simulink model "Final_Model_Building_2_AirflowAdded"  (R2022a)
settings: Solver=ode1  StartTime=0.0  StopTime=24*3600  FixedStep=10  RelTol=1e-3
values from neighbouring files (symbols this model uses):
  Aux_Threshold = 52    [Setup_Code_EWASP_VC.m]
  buildingAge = 2005    [Setup_Code_EWASP_VC.m]
  ceilingHeight = 2.4    [Setup_Code_EWASP_VC.m]
  conductiveHconnectMatrix = [ ... (first row only)    [Setup_Code_EWASP_VC.m]
  cRoofGreen = 100000    [Setup_Code_EWASP_VC.m]
  Defrost_After_Time = 30    [Setup_Code_EWASP_VC.m]
  DHWDemandProfile = occFreegainHotwaterElecTestPassiveOcc3(:,3)    [Setup_Code_EWASP_VC.m]
  Elec_Max = Elec_Max*(30/24.2)    [Setup_Code_EWASP_VC.m]
  Elec_Mid = Elec_Mid*(30/24.2)    [Setup_Code_EWASP_VC.m]
  Elec_Min = Elec_Min*(30/24.2)    [Setup_Code_EWASP_VC.m]
  ElecDemandProfile = occFreegainHotwaterElecTestPassiveOcc3(:,4)    [Setup_Code_EWASP_VC.m]
  ElecFixed = [Elec_Max(6,2) Elec_Max(6,4) Elec_Max(6,6) Elec_Max(6,7) ... (first row only)    [Setup_Code_EWASP_VC.m]
  floorOrCeilingArea = floorOrCeilingArea*1.15    [Setup_Code_EWASP_VC.m]
  forceCold = 0    [Setup_Code_EWASP_VC.m]
  freegain = occFreegainHotwaterElecTestPassiveOcc3(:,2)-max(occupancy)*25    [Setup_Code_EWASP_VC.m]
  furnitureModelOn = 1    [Setup_Code_EWASP_VC.m]
  Heat_Max = Heat_Max*(30/24.2)    [Setup_Code_EWASP_VC.m]
  Heat_Mid = Heat_Mid*(30/24.2)    [Setup_Code_EWASP_VC.m]
  Heat_Min = Heat_Min*(30/24.2)    [Setup_Code_EWASP_VC.m]
  HeatFixed = [Heat_Max(6,2) Heat_Max(6,4) Heat_Max(6,6) Heat_Max(6,7) ... (first row only)    [Setup_Code_EWASP_VC.m]
  HeatingOnProfile = repmat(HeatingOnProfile,365,1)    [Setup_Code_EWASP_VC.m]
  HEX_ReturnLowerLimit = 52.5    [Setup_Code_EWASP_VC.m]
  HEX_ReturnUpperLimit = 55    [Setup_Code_EWASP_VC.m]
  LeakMultiplier = 1+(2*(rand()-0.5)/10)    [Setup_Code_EWASP_VC.m]
  maxOcc = max(occupancyProfile)    [Setup_Code_EWASP_VC.m]
  NESW_wallArea = max(NESW_Lengths*ceilingHeight-NESW_Windows,0)    [Setup_Code_EWASP_VC.m]
  NESW_Windows = [ ... (first row only)    [Setup_Code_EWASP_VC.m]
  numRooms = roomCount    [Setup_Code_EWASP_VC.m]
  occupancy = occupancyProfile    [Setup_Code_EWASP_VC.m]
  offsetDays = 0    [Setup_Code_EWASP_VC.m]
  pumpChoice = pumpChoices(MinIndex,1)    [Setup_Code_EWASP_VC.m]
  pumpRamp = 180    [Setup_Code_EWASP_VC.m]
  ReturnLowerLimit = 37.5    [Setup_Code_EWASP_VC.m]
  ReturnUpperLimit = 40    [Setup_Code_EWASP_VC.m]
  RoofIrradiance = Flat_NS_EW_RoofIrradiance(:,1)    [Setup_Code_EWASP_VC.m]
  roofStartTemp = ones(11,1)*20    [Setup_Code_EWASP_VC.m]
  rooftype = 0    [Setup_Code_EWASP_VC.m]
  RoomDataMatrix = [zeros(1,12);ones(1,12)*wallDensity;zeros(1,12);ones(1,12)*wallU;ones(1,12)*windowU;ones(1,12)*floorU;ones(1,12)*ceilingU;zeros(1,12);windowArea, 0;floorOrCeilingArea;zeros(1,12);floorOrCeilingArea*ceilingHeight]    [Setup_Code_EWASP_VC.m]
  roomVol = roomVol*1.15    [Setup_Code_EWASP_VC.m]
  slabStartTemp = (GroundTempTimeSeries(offsetDays*1440+1,1)+thermostatSetting)/2    [Setup_Code_EWASP_VC.m]
  SlackRequest = zeros(1440,1)    [Setup_Code_EWASP_VC.m]
  SolarThermalExists = 0    [Setup_Code_EWASP_VC.m]
  SourceFixed = HeatFixed-ElecFixed    [Setup_Code_EWASP_VC.m]
  StateSeries = StateSeriesGenerator(22,7,1)    [Setup_Code_EWASP_VC.m]
  Tank_Lower_Temp = 49.5    [Setup_Code_EWASP_VC.m]
  Tank_Upper_Temp = 52    [Setup_Code_EWASP_VC.m]
  Tank_Volume_m3 = 0.15    [Setup_Code_EWASP_VC.m]
  TankHeatHour = randi([1 5])-1    [Setup_Code_EWASP_VC.m]
  upDown = [0;0;0;0;1;1;1;1;1;1;1]    [Setup_Code_EWASP_VC.m]
  wallStartTempExt = thermostatSetting*(0.266+0.00215*outdoorStartTemp+0.018*wallU+0.00113*outdoorStartTemp*wallU+0.0068*wallU^2)    [Setup_Code_EWASP_VC.m]
undefined symbols (not defined in the file or in its folder): a, ceilingU, condUDMatrix, convUDMatrix, deltaPEXPANDED_E, deltaPEXPANDED_E2, deltaPEXPANDED_N, deltaPEXPANDED_N2, deltaPEXPANDED_S, deltaPEXPANDED_S2, deltaPEXPANDED_W, deltaPEXPANDED_W2, DesiredDHWTemp, DesiredFlowTempVsInOutDeltaTemp, DiffuseHorizontal, DiscIntNeverNeededParam, DNI, dwnAndConcrete, DWORK_A_HX, DWORK_CHK_FLU, DWORK_CP_NODE, DWORK_DH, DWORK_FLUID, DWORK_HCON, DWORK_LOSS, DWORK_MDOTDOWN, DWORK_MDOTIN, DWORK_MDOTUP, DWORK_MIX, DWORK_PRESS, DWORK_QDOTIN, DWORK_RHO_NODE, DWORK_TIN, DWORK_TS_OLD, DWORK_V_NODE, ExtractRates, GroundTempTimeSeries, HCM, HCM2, HCM_closed, HCM_closed2, intermediateU, IsTop, massFlowMatrix, mechEfficiency, neighbourMatrix, numericalRoomUse, RadiatorMatrix, room2roomflowmatrix_E, room2roomflowmatrix_E2, room2roomflowmatrix_N, room2roomflowmatrix_N2, room2roomflowmatrix_S, room2roomflowmatrix_S2, room2roomflowmatrix_W, room2roomflowmatrix_W2, StateAirInEXPANDED_E, StateAirInEXPANDED_E2, StateAirInEXPANDED_N, StateAirInEXPANDED_N2 ... (+27)
libraries: simulink x6, dspsigops x4, dspmtrx3 x4, carnot x3, spsEdgeDetectorLib x2, dspstat3 x2, powerlib_meascontrol x1, simulink_extras x1
(part 12 of 27)

== system Final_Model_Building_2_AirflowAdded/ASHP_Subsystem/DHW for ASHP Case/Storage_Type_2_CONF ==
  note: upper heat exchanger (backup heater)
  note: pipe connection for DHW
  note: pipe connection for DHW circulation
  Tamb : Inport
  Temp_HX : Inport  Port=2
  THB_dhw : Inport  Port=3
  THB_circ : Inport  Port=4
  Mdot_dhw1 : Inport  Port=5
  Mdot_dhw2 : Inport  Port=6
  mdotHEX : Inport  Port=7
  HX_EN12977_1 : Subsystem  AncestorBlock=carnot/Storage/Thermal/Storage_Ports/HX_EN12977  mask(heat exchanger for storage, data EN 12977){h_in=hx1inlet, h_out=hx1outlet, hgt=hgt, dia=hx1dia, height=-0.68756, ua0=hx1uac, uam=hx1uam, uat=hx1uat, dpqua=hx1dpqua, nodes=nodes}
      mask prompts: h_in "relative height of inlet"; h_out "relative height of outlet"; hgt "Height of storage in m"; dia "Diameter of HX pipe [m]"; height "Height difference inlet-outlet [m]"; ua0 "uac: heat transfer coefficient [W/K /(kg/s) /(°C)]"; uam "uam: massflow dependent heat transfer [-]"; uat "uat: temperature difference dependent heat transfer [-]"; dpqua "Pressure drop coefficient dpqua [Pa/(kg/s)²]"; nodes "number of nodes"
      mask help:
      | The block transforms the incoming THV vector to a vector which the storage interprets as a heat exchanger.
      | Give inlet and outlet as a relative position 0=bottom to 1=top
      | The heat transfer is calculated by:
      | UA = uac * mdot^uam * ((Theatexchanger+Tstorage)/2)^uat
      mask init:
      | in = zeros(nodes,1);    % vector of length nodes
      | up = in;                % vector of length nodes
      | down = in;              % vector of length nodes
      | 
      | h_in = max(0,h_in);     % no nodes below 0
      | h_out = max(0,h_out);   % no nodes below 0
      | 
      | inlet = round(h_in*(nodes-1))+1;    % inlet position
      | outlet = round(h_out*(nodes-1))+1;  % outlet position
      | set_param(gcb,'height',num2str((h_out-h_in)*hgt));
      | % hgt = (h_out-h_in)*hgt;
      | 
      | in(inlet)=1;
      | 
      | if (h_in < h_out)           % if inlet below outlet
      |     up(inlet:outlet)=1;     % upwards
      | elseif (h_in > h_out)       % else if inlet above outlet
      |     down(outlet:inlet)=1;   % downwards
      | end
      mask Help: web(['file:///' fullfile(path_carnot('help'),'StoragePorts_HeatExchangerModels.html')],'-helpbrowser')
      mask TypeOptions dia: Pressure_Drop_StorageHX/dia
      mask TypeOptions height: Pressure_Drop_StorageHX/hgt
      mask TypeOptions ua0: sfun_storage_heatexchanger/p1
      mask TypeOptions uam: sfun_storage_heatexchanger/p2
      mask TypeOptions uat: sfun_storage_heatexchanger/p3
      mask TypeOptions dpqua: Pressure_Drop_StorageHX/dpqua
      mask TypeOptions nodes: sfun_storage_heatexchanger/nodes
      mask DialogControl ParameterTabVar0 Prompt: Geometry
      mask DialogControl ParameterTabVar01 Prompt: Heat transfer
      mask DialogControl ParameterTabVar012 Prompt: Pressure drop
      mask DialogControl ParameterTabVar0123 Prompt: Calculation
      mask Display: disp('HX EN12977')
  Mux : Mux  Inputs=2
  Mux1 : Mux  Inputs=2
  Pipe_Connection_1 : Subsystem  AncestorBlock=carnot/Storage/Thermal/Storage_Ports/Pipe_Connection  mask(pipe connection to storage){h_in=pipe1inlet, h_out=pipe1outlet, hgt=hgt, nodes=nodes}
      mask prompts: h_in "relative height of inlet, range from 0 (= bottom) to 1 (= top)"; h_out "relative height of outlet, range from 0 (= bottom) to 1 (= top)"; hgt "Height of storage in m"; nodes "Number of nodes of storage (DO NOT CHANGE)"
      mask help: The block transforms the incoming THV vector to a vector which the storage interprets as a flow into the storage fluid.
      mask init:
      | in = zeros(nodes,1);    % vector of length nodes
      | up = in;                % vector of length nodes
      | down = in;              % vector of length nodes
      | 
      | h_in = max(0,min(h_in,1));     % no nodes below 0
      | h_out = max(0,min(h_out,1));   % no nodes below 0
      | %set_param(gcb,'height',num2str((h_out-h_in)*hgt));
      |  
      | inlet = max(ceil(h_in*nodes),1);    % inlet position
      | outlet = max(ceil(h_out*nodes),1);  % outlet position
      |  
      | in(inlet)=1;
      |  
      | idx_in_out = inlet:outlet;
      | if (inlet < outlet)         % if inlet below outlet
      |     up(inlet:outlet-1)=1;   % upwards
      | elseif (inlet > outlet)     % else if inlet above outlet
      |     down(outlet:inlet-1)=1; % downwards
      |     idx_in_out = outlet:inlet;
      | end
      mask Help: web(fullfile(path_carnot('help'),'StoragePorts_PipeConnections.html'),'-helpbrowser')
      mask DialogControl ParameterTabVar0 Prompt: Geometry
      mask DialogControl ParameterTabVar02 Prompt: Calulation
      mask Display: disp('Pipe')
  Pipe_Connection_2 : Subsystem  AncestorBlock=carnot/Storage/Thermal/Storage_Ports/Pipe_Connection  mask(pipe connection to storage){h_in=pipe2inlet, h_out=pipe2outlet, hgt=hgt, nodes=nodes}
      mask prompts: h_in "relative height of inlet, range from 0 (= bottom) to 1 (= top)"; h_out "relative height of outlet, range from 0 (= bottom) to 1 (= top)"; hgt "Height of storage in m"; nodes "Number of nodes of storage (DO NOT CHANGE)"
      mask help: The block transforms the incoming THV vector to a vector which the storage interprets as a flow into the storage fluid.
      mask init: same as Final_Model_Building_2_AirflowAdded/ASHP_Subsystem/DHW for ASHP Case/Storage_Type_2_CONF/Pipe_Connection_1
      mask Help: web(fullfile(path_carnot('help'),'StoragePorts_PipeConnections.html'),'-helpbrowser')
      mask DialogControl ParameterTabVar0 Prompt: Geometry
      mask DialogControl ParameterTabVar02 Prompt: Calulation
      mask Display: disp('Pipe')
  Scope : Scope
  Scope1 : Scope
  Scope2 : Scope
  T_Sensor_Surface : carnot/Control/T_Sensor_Surface  pos=Tsensor  tdel=10  t0=mean(tini)
      settings: SourceProductName=Carnot
  Terminator1 : Terminator
  sfun_storageTnodesjh : S-Function  AncestorBlock=carnot/Basic/Thermal_Models/sfun_storageTnodes  FunctionName=storage_TnodesMOD  Parameters=dia, volume, standing, uloss , ubot, utop, cond, tini, nodes, nconnect, elimthermocline, condinvtc  SFunctionDeploymentMode=off  EnableBusSupport=off  SFcnStateName=DWORK_DH  mask(sfunction storage_Tnodes){uloss=uwall, ubot=ubot, utop=utop, cond=axcond, volume=volume, dia=dia, standing=standing cylinder, tini=tini, nodes=nodes, nconnect=3, elimthermocline=1, condinvtc=1e5}
      mask prompts: uloss "Heat transfer coefficient to ambient [W/m²K]"; ubot "Heat transfer coefficient to ambient bottom [W/m²K]"; utop "Heat transfer coefficient to ambient top [W/m²K]"; cond "Effective thermal conductivity [W/m/K]"; volume "Volume [m³]"; dia "Diameter [m]"; standing "Position"; tini "Initial temperature in °C"; nodes "Number of nodes"; nconnect "Number of ports"; elimthermocline "Elimination method (0 = off, 1 = temperature dependant, 2 = density dependant)"; condinvtc "COND_ITC: heat transport coefficient for the method 2"
      mask help:
      | The differential equation is derived from the energy conservation equation by using the finite volume method [Patankar: Numerical Heat Transfer and Fluid Flow, 1980].
      | Methods to eliminate the inversed thermocline (It occurs when node with lower density is below a node with higher density. Typically it can be translated to a node with higher temperature below a node with lower temperature. Exception is water below 4°C.):
      | 0 - inversed thermocline is not eliminated
      | 1 - Temperature based: An inversed thermocline exists , if the  temperature of the lower node is more than LIMIT_T_INVERSED degrees  above the upper node. In that case the temperatures of the nodes are mixed. For the geometry of a laying cylinder the different volumes of the nodes are taken in account.
      |  2 - Density based : An inversed thermocline exists, if the density of the lower node is less than the density of the upper node. The model  adds an additional heat transport towards the upper node:
      | heat transport [W/m³] = COND_ITC[W*m³/kg] * density_differnce[kg/m³] / node[m³]
      mask init:
      | if isempty(uloss)
      |     uloss = 1;
      | end
      | 
      | if isempty(ubot)
      |     ubot = 1;
      | end
      | 
      | if isempty(utop)
      |     utop = 1;
      | end
      | 
      | if isempty(cond)
      |     cond = 1;
      | end
      | 
      | if isempty(volume)
      |     volume = 1;
      | end
      | 
      | if isempty(dia)
      |     dia = 1;
      | end
      | 
      | if isempty(standing)
      |     standing = 1;
      | end
      | 
      | if numel(tini) ~= nodes
      |     tini = 20*ones(1,nodes);
      | end
      | 
      | if isempty(nodes)
      |     nodes = 200;
      | end
      | 
      | if isempty(nconnect)
      |     nconnect = 10;
      | end
      | 
      | if isempty(elimthermocline)
      |     elimthermocline = 2;
      | end
      | 
      | if isempty(condinvtc)
      |     condinvtc = 1e5;
      | end
      mask Help: web(fullfile(path_carnot('help'),'Storage_Type_N.html'),'-helpbrowser')
      mask TypeOptions standing: standing cylinder | lying cylinder
      mask DialogControl Container5 Prompt: Thermal
      mask DialogControl Container6 Prompt: Geometry
      mask DialogControl Container7 Prompt: Caclulation
      mask DialogControl Container10 Prompt: Inversed thermocline
      mask Display:
      | disp('storage_Tnodes')
      | 
      | port_label('input', 1, 'Tamb')
      | port_label('output', 1, 'Energy')
      | port_label('output', 2, 'Tnodes')
      | 
      | if exist('nconnect','var')
      |     for n = 1:nconnect
      |         port_label('input',  n+1, ['port' num2str(n)])
      |     end
      | end
  Tsensors : Outport  VectorParamsAs1DForOutWhenUnconnected=off
  THB_hx : Outport  Port=2  VectorParamsAs1DForOutWhenUnconnected=off
  THBdhw : Outport  Port=3  VectorParamsAs1DForOutWhenUnconnected=off
  AuxHeat : Outport  Port=4  VectorParamsAs1DForOutWhenUnconnected=off
  wires:
  HX_EN12977_1/1(to_storeT) -> sfun_storageTnodesjh/4
  Pipe_Connection_2/1(to_storeT) -> Scope/1, sfun_storageTnodesjh/3
  THB_circ/1 -> Mux1/1  "THBinPipe2"
  Tamb/1 -> sfun_storageTnodesjh/1  "Tamb"
  sfun_storageTnodesjh/2 -> Scope2/1, T_Sensor_Surface/1, HX_EN12977_1/1(from_storeT)  "Tnodes"
  Pipe_Connection_1/1(to_storeT) -> THBdhw/1, sfun_storageTnodesjh/2, Scope1/1
  Temp_HX/1 -> HX_EN12977_1/2(Tempin)
  HX_EN12977_1/2(TempHEXout) -> THB_hx/1
  T_Sensor_Surface/1 -> Tsensors/1
  Mdot_dhw1/1 -> Mux/2  "THBinPipe1"
  sfun_storageTnodesjh/1 -> Terminator1/1  "Energy"
  Mdot_dhw2/1 -> Mux1/2  "THBinPipe1"
  THB_dhw/1 -> Mux/1  "THBinPipe1"
  Mux/1 -> Pipe_Connection_1/1(THBin)
  Mux1/1 -> Pipe_Connection_2/1(THBin)
  mdotHEX/1 -> HX_EN12977_1/3(massFlowIn)
  HX_EN12977_1/3(AuxHeat) -> AuxHeat/1

== system Final_Model_Building_2_AirflowAdded/ASHP_Subsystem/DHW for ASHP Case/Subsystem ==
  In1 : Inport
  Ceil : Rounding
  Constant1 : Constant  Value=60
  Constant2 : Constant  Value=60
  Digital Clock : DigitalClock  SampleTime=10
  Direct Lookup Table (n-D) : LookupNDDirect  NumberOfTableDimensions=1  TableIsInput=on
  Divide : Product  Inputs=*/
  Divide1 : Product  Inputs=*/
  Saturation : Saturate  UpperLimit=1440*365  LowerLimit=0
  Out1 : Outport  VectorParamsAs1DForOutWhenUnconnected=off
  wires:
  Divide1/1 -> Direct Lookup Table (n-D)/2
  Divide/1 -> Ceil/1
  Digital Clock/1 -> Divide/1
  Constant1/1 -> Divide/2
  In1/1 -> Divide1/1
  Direct Lookup Table (n-D)/1 -> Out1/1
  Constant2/1 -> Divide1/2
  Ceil/1 -> Saturation/1
  Saturation/1 -> Direct Lookup Table (n-D)/1

== system Final_Model_Building_2_AirflowAdded/ASHP_Subsystem/DHW for ASHP Case/Switch Case Action Subsystem ==
  In1 : Inport
  Action Port : ActionPort  ActionPortLabel=default:
  1 m : Relay  OnSwitchValue=Tank_Upper_Temp  OffSwitchValue=Tank_Lower_Temp  OnOutputValue=0  OffOutputValue=1  OutDataTypeStr=boolean
  Out1 : Outport  VectorParamsAs1DForOutWhenUnconnected=off
  wires:
  In1/1 -> 1 m/1
  1 m/1 -> Out1/1

== system Final_Model_Building_2_AirflowAdded/ASHP_Subsystem/DHW for ASHP Case/Switch Case Action Subsystem1 ==
  In1 : Inport
  Action Port : ActionPort  ActionPortLabel=case [ 0 ]:
  'Aux Required' Alternative1 : Relay  OnSwitchValue=Aux_Threshold  OffSwitchValue=Aux_Threshold-0.1  OnOutputValue=0  OffOutputValue=1  OutDataTypeStr=boolean
  Out1 : Outport  VectorParamsAs1DForOutWhenUnconnected=off
  wires:
  In1/1 -> 'Aux Required' Alternative1/1
  'Aux Required' Alternative1/1 -> Out1/1

== system Final_Model_Building_2_AirflowAdded/ASHP_Subsystem/DHW for ASHP Case/Switch Case Action Subsystem2 ==
  In1 : Inport
  Action Port : ActionPort  ActionPortLabel=default:
  1 means tank temp recently fell below 49.1 : Relay  OnSwitchValue=60  OffSwitchValue=49.5  OnOutputValue=0  OffOutputValue=1  OutDataTypeStr=boolean
  Out1 : Outport  VectorParamsAs1DForOutWhenUnconnected=off
  wires:
  In1/1 -> 1 means tank temp recently fell below 49.1/1
  1 means tank temp recently fell below 49.1/1 -> Out1/1

== system Final_Model_Building_2_AirflowAdded/ASHP_Subsystem/DHW for ASHP Case/Switch Case Action Subsystem3 ==
  In1 : Inport
  Action Port : ActionPort  ActionPortLabel=case [ 0 ]:
  'Aux Required' Alternative : Relay  OnSwitchValue=60  OffSwitchValue=Aux_Threshold  OnOutputValue=0  OffOutputValue=1  OutDataTypeStr=boolean
  Out1 : Outport  VectorParamsAs1DForOutWhenUnconnected=off
  wires:
  In1/1 -> 'Aux Required' Alternative/1
  'Aux Required' Alternative/1 -> Out1/1

== system Final_Model_Building_2_AirflowAdded/ASHP_Subsystem/Defrost Timer/Subsystem ==
  In1 : Inport
  In2 : Inport  Port=2
  1-D Lookup Table : Lookup_n-D  NumberOfTableDimensions=1  BreakpointsForDimension1=[-9.9 1.69 1.71 10]  Table=[0.1833 0.1157 0 0]  InternalRulePriority=Speed  RndMeth=Simplest
  Add One seconds worth of half an hour : Constant
  Add Zero : Constant  Value=0
  Add Zero1 : Constant  Value=10
  Add Zero2 : Constant  Value=0
  Display : Display
  Divide : Product  Inputs=*/
  Divide1 : Product  Inputs=**
  Do Nothing : Constant  Value=0
  Integrator : Integrator  ExternalReset=rising  ShowStatePort=on
  Integrator1 : Integrator  ExternalReset=rising
  Logical Operator : Logic  AllPortsSameDT=off  OutDataTypeStr=boolean
  Relational Operator : RelationalOperator  Operator=<=  OutDataTypeStr=boolean  RndMeth=Simplest  InputSameDT=off
  Reset Integrator : Constant
  Reset Integrator1 : Constant
  Sample and Hold : dspsigops/Sample and Hold  trig=Rising edge  initCond=240  latchinput=on
  Scope1 : Scope
  Scope2 : Scope
  Scope3 : Scope
  Switch{,1..3} (4 alike) : Switch  Threshold=1  SaturateOnIntegerOverflow=off  InputSameDT=off
  Temperature2 : Constant  Value=1.7
  minutes of cold operation before defrost : Constant  Value=Defrost_After_Time
  seconds in 1 min : Constant  Value=60
  Out1 : Outport  VectorParamsAs1DForOutWhenUnconnected=off
  Out2 : Outport  Port=2  VectorParamsAs1DForOutWhenUnconnected=off
  Out3 : Outport  Port=3  VectorParamsAs1DForOutWhenUnconnected=off
  wires:
  In1/1 -> Switch2/1, Relational Operator/1
  Integrator/State -> Switch1/2
  In2/1 -> Switch3/2
  Relational Operator/1 -> Logical Operator/1
  Integrator1/1 -> Sample and Hold/1, Scope1/1
  Switch1/1 -> Integrator/2, Scope3/1, Out1/1, Sample and Hold/Trigger, Integrator1/2
  Switch2/1 -> 1-D Lookup Table/1
  Add One seconds worth of half an hour/1 -> Divide/1
  Integrator/1 -> Scope2/1, Out3/1, Display/1
  Temperature2/1 -> Relational Operator/2
  Switch/1 -> Integrator/1
  Add Zero1/1 -> Switch2/3
  Reset Integrator1/1 -> Switch3/1
  Do Nothing/1 -> Switch1/3
  Logical Operator/1 -> Switch/2, Switch2/2
  Switch3/1 -> Logical Operator/2
  Add Zero2/1 -> Switch3/3
  Reset Integrator/1 -> Switch1/1
  Add Zero/1 -> Switch/3
  1-D Lookup Table/1 -> Integrator1/1
  Sample and Hold/1 -> Out2/1
  Divide1/1 -> Divide/2
  Divide/1 -> Switch/1
  seconds in 1 min/1 -> Divide1/2
  minutes of cold operation before defrost/1 -> Divide1/1

== system Final_Model_Building_2_AirflowAdded/ASHP_Subsystem/Defrost Timer/Subsystem1 ==
  In1 : Inport
  In2 : Inport  Port=2
  In3 : Inport  Port=3
  Counter On? (i.e. not currently defrosting?)1 : Constant  Value=0
  Counter On? (i.e. not currently defrosting?)3 : Constant  Value=20
  Discrete-Time Integrator : DiscreteIntegrator  gainval=1  ExternalReset=rising  SampleTime=-1  ICPrevOutput=DiscIntNeverNeededParam  ICPrevScaledInput=DiscIntNeverNeededParam
  Integrator1 : Integrator  ExternalReset=rising  ShowStatePort=on
  Product : Product  Inputs=*/
  Product2 : Product
  Saturation : Saturate  UpperLimit=1  LowerLimit=0
  Switch : Switch  Threshold=1  SaturateOnIntegerOverflow=off  InputSameDT=off
  Terminator : Terminator
  Terminator1 : Terminator
  "d " : Constant
  Out1 : Outport  VectorParamsAs1DForOutWhenUnconnected=off
  wires:
  "d "/1 -> Switch/1
  Product/1 -> Switch/2
  Discrete-Time Integrator/1 -> Product2/1
  Switch/1 -> Discrete-Time Integrator/2, Integrator1/2
  Counter On? (i.e. not currently defrosting?)1/1 -> Switch/3
  In2/1 -> Product/2
  In1/1 -> Discrete-Time Integrator/1
  Counter On? (i.e. not currently defrosting?)3/1 -> Product2/2
  Product2/1 -> Saturation/1
  Saturation/1 -> Out1/1, Integrator1/1
  Integrator1/State -> Product/1
  Integrator1/1 -> Terminator/1
  In3/1 -> Terminator1/1

== system Final_Model_Building_2_AirflowAdded/ASHP_Subsystem/Subsystem14/HeatPump_Simplified ==
  THBsource : Inport
  THB_r : Inport  Port=2
  Tamb : Inport  Port=3
  Ctrl : Inport  Port=4
  mdot_cold : Inport  Port=5
  mdot_hot : Inport  Port=6
  Defrost Delta In : Inport  Port=7
  Defrost Delta In1 : Inport  Port=8
  HeatPump_basic : Subsystem  AncestorBlock=carnot/Basic/Thermal_Models/HeatPump_basic  mask(heat pump){K=K, caph=caph, capc=capc, UA=UA}
      mask prompts: K "Parameters K (see also HP_param.m)"; caph "thermal capacity hot loop [J/K]"; capc "thermal capacity cold loop [J/K]"; UA "heat loss coefficient [W/K]"
      mask help:
      | Linearized heat pump model, uses measured data according to EN 14511 as input (Schwamberger, K.: Fortschrittsberichete VDI, Nr. 263, 1991).
      | heating power: Qdot_h = K1*Tcold_in + K2*Thot_out + K3
      | electric power: Pel = K4*Tcold_in + K5*Thot_out + K6
      | source power: Qdot_c = -K7*Tcold_in - K8*Thot_out - K9
      | differential equation: cap*dTh/dt = Qdot + mdot*cp*(T_in-T) + UA*(Tamb-T)
      | with: cap = mass * heat_capactiy
      | See hp_param.m for the parameters K1 to K9.
      mask Help: web(fullfile(path_carnot('help'),'HeatPump_basic.html'),'-helpbrowser')
      mask DialogControl ParameterTabVar0 Prompt: HP Caracteristic
      mask DialogControl ParameterTabVar01 Prompt: Thermal
      mask Display: plot(0,-30,120,130,[30,46,36,46,36,46,30],[40,40,50,60,70,80,80],[70,54,64,54,64,54,64,54,64,54,70],[40,40,44,50,55,60,65,70,75,80,80],[56,45],[95,95],[51,51],[82,95])
  T_source : Outport  VectorParamsAs1DForOutWhenUnconnected=off
  "T_out " : Outport  Port=2  VectorParamsAs1DForOutWhenUnconnected=off
  HPdat : Outport  Port=3  VectorParamsAs1DForOutWhenUnconnected=off
  Real P_Therm : Outport  Port=4  VectorParamsAs1DForOutWhenUnconnected=off
  Main Delta : Outport  Port=5  VectorParamsAs1DForOutWhenUnconnected=off
  wires:
  HeatPump_basic/2(THBload) -> "T_out "/1  "THB_s"
  THBsource/1 -> HeatPump_basic/1(Tin_cold)
  THB_r/1 -> HeatPump_basic/2(Tin_hot)
  Tamb/1 -> HeatPump_basic/3(Tamb)
  Ctrl/1 -> HeatPump_basic/4(Ctrl)
  HeatPump_basic/1(Tsource) -> T_source/1  "THBsource"
  HeatPump_basic/3(HPdat) -> HPdat/1
  HeatPump_basic/4(Real P_Therm) -> Real P_Therm/1
  mdot_cold/1 -> HeatPump_basic/5(mdot_in_cold)
  mdot_hot/1 -> HeatPump_basic/6(mdot_in_hot)
  HeatPump_basic/5(Main Delta) -> Main Delta/1
  Defrost Delta In/1 -> HeatPump_basic/7(Defrost Delta In)
  Defrost Delta In1/1 -> HeatPump_basic/8(Ctrl1)

== system Final_Model_Building_2_AirflowAdded/ASHP_Subsystem/Subsystem14/HeatPump_Simplified1 ==
  THBsource : Inport
  THB_r : Inport  Port=2
  Tamb : Inport  Port=3
  Ctrl : Inport  Port=4
  mdot_cold : Inport  Port=5
  mdot_hot : Inport  Port=6
  Main Delta In : Inport  Port=7
  HeatPump_basic : Subsystem  AncestorBlock=carnot/Basic/Thermal_Models/HeatPump_basic  mask(heat pump){K=K, caph=caph, capc=capc, UA=UA}
      mask prompts: K "Parameters K (see also HP_param.m)"; caph "thermal capacity hot loop [J/K]"; capc "thermal capacity cold loop [J/K]"; UA "heat loss coefficient [W/K]"
      mask help:
      | Linearized heat pump model, uses measured data according to EN 14511 as input (Schwamberger, K.: Fortschrittsberichete VDI, Nr. 263, 1991).
      | heating power: Qdot_h = K1*Tcold_in + K2*Thot_out + K3
      | electric power: Pel = K4*Tcold_in + K5*Thot_out + K6
      | source power: Qdot_c = -K7*Tcold_in - K8*Thot_out - K9
      | differential equation: cap*dTh/dt = Qdot + mdot*cp*(T_in-T) + UA*(Tamb-T)
      | with: cap = mass * heat_capactiy
      | See hp_param.m for the parameters K1 to K9.
      mask Help: web(fullfile(path_carnot('help'),'HeatPump_basic.html'),'-helpbrowser')
      mask DialogControl ParameterTabVar0 Prompt: HP Caracteristic
      mask DialogControl ParameterTabVar01 Prompt: Thermal
      mask Display: plot(0,-30,120,130,[30,46,36,46,36,46,30],[40,40,50,60,70,80,80],[70,54,64,54,64,54,64,54,64,54,70],[40,40,44,50,55,60,65,70,75,80,80],[56,45],[95,95],[51,51],[82,95])
  T_source : Outport  VectorParamsAs1DForOutWhenUnconnected=off
  "T_out " : Outport  Port=2  VectorParamsAs1DForOutWhenUnconnected=off
  HPdat : Outport  Port=3  VectorParamsAs1DForOutWhenUnconnected=off
  Real P_Therm : Outport  Port=4  VectorParamsAs1DForOutWhenUnconnected=off
  Defrost Delta : Outport  Port=5  VectorParamsAs1DForOutWhenUnconnected=off
  wires:
  HeatPump_basic/2(THBload) -> "T_out "/1  "THB_s"
  THBsource/1 -> HeatPump_basic/1(Tin_cold)
  THB_r/1 -> HeatPump_basic/2(Tin_hot)
  Tamb/1 -> HeatPump_basic/3(Tamb)
  Ctrl/1 -> HeatPump_basic/4(Ctrl)
  HeatPump_basic/1(Tsource) -> T_source/1  "THBsource"
  HeatPump_basic/3(HPdat) -> HPdat/1
  HeatPump_basic/4(Real P_Therm) -> Real P_Therm/1
  mdot_cold/1 -> HeatPump_basic/5(mdot_in_cold)
  mdot_hot/1 -> HeatPump_basic/6(mdot_in_hot)
  HeatPump_basic/5(Defrost Delta) -> Defrost Delta/1
  Main Delta In/1 -> HeatPump_basic/7(Main Delta In)

== system Final_Model_Building_2_AirflowAdded/ASHP_Subsystem_Variable/DHW for ASHP Case/HeatPump_Simplified1 ==
  THBsource : Inport
  THB_r : Inport  Port=2
  Tamb : Inport  Port=3
  Ctrl : Inport  Port=4
  mdot_cold : Inport  Port=5
  mdot_hot : Inport  Port=6
  Main Delta In : Inport  Port=7
  HeatPump_basic : Subsystem  AncestorBlock=carnot/Basic/Thermal_Models/HeatPump_basic  mask(heat pump){K=K, caph=caph, capc=capc, UA=UA}
      mask prompts: K "Parameters K (see also HP_param.m)"; caph "thermal capacity hot loop [J/K]"; capc "thermal capacity cold loop [J/K]"; UA "heat loss coefficient [W/K]"
      mask help:
      | Linearized heat pump model, uses measured data according to EN 14511 as input (Schwamberger, K.: Fortschrittsberichete VDI, Nr. 263, 1991).
      | heating power: Qdot_h = K1*Tcold_in + K2*Thot_out + K3
      | electric power: Pel = K4*Tcold_in + K5*Thot_out + K6
      | source power: Qdot_c = -K7*Tcold_in - K8*Thot_out - K9
      | differential equation: cap*dTh/dt = Qdot + mdot*cp*(T_in-T) + UA*(Tamb-T)
      | with: cap = mass * heat_capactiy
      | See hp_param.m for the parameters K1 to K9.
      mask Help: web(fullfile(path_carnot('help'),'HeatPump_basic.html'),'-helpbrowser')
      mask DialogControl ParameterTabVar0 Prompt: HP Caracteristic
      mask DialogControl ParameterTabVar01 Prompt: Thermal
      mask Display: plot(0,-30,120,130,[30,46,36,46,36,46,30],[40,40,50,60,70,80,80],[70,54,64,54,64,54,64,54,64,54,70],[40,40,44,50,55,60,65,70,75,80,80],[56,45],[95,95],[51,51],[82,95])
  T_source : Outport  VectorParamsAs1DForOutWhenUnconnected=off
  "T_out " : Outport  Port=2  VectorParamsAs1DForOutWhenUnconnected=off
  HPdat : Outport  Port=3  VectorParamsAs1DForOutWhenUnconnected=off
  Real P_Therm : Outport  Port=4  VectorParamsAs1DForOutWhenUnconnected=off
  Defrost Delta : Outport  Port=5  VectorParamsAs1DForOutWhenUnconnected=off
  wires:
  HeatPump_basic/2(THBload) -> "T_out "/1  "THB_s"
  THBsource/1 -> HeatPump_basic/1(Tin_cold)
  THB_r/1 -> HeatPump_basic/2(Tin_hot)
  Tamb/1 -> HeatPump_basic/3(Tamb)
  Ctrl/1 -> HeatPump_basic/4(Ctrl)
  HeatPump_basic/1(Tsource) -> T_source/1  "THBsource"
  HeatPump_basic/3(HPdat) -> HPdat/1
  HeatPump_basic/4(Real P_Therm) -> Real P_Therm/1
  mdot_cold/1 -> HeatPump_basic/5(mdot_in_cold)
  mdot_hot/1 -> HeatPump_basic/6(mdot_in_hot)
  HeatPump_basic/5(Defrost Delta) -> Defrost Delta/1
  Main Delta In/1 -> HeatPump_basic/7(Main Delta In)

== system Final_Model_Building_2_AirflowAdded/ASHP_Subsystem_Variable/DHW for ASHP Case/HeatPump_Simplified2 ==
  THBsource : Inport
  THB_r : Inport  Port=2
  Tamb : Inport  Port=3
  Ctrl : Inport  Port=4
  mdot_cold : Inport  Port=5
  mdot_hot : Inport  Port=6
  Defrost Delta In : Inport  Port=7
  HeatPump_basic : Subsystem  AncestorBlock=carnot/Basic/Thermal_Models/HeatPump_basic  mask(heat pump){K=K, caph=caph, capc=capc, UA=UA}
      mask prompts: K "Parameters K (see also HP_param.m)"; caph "thermal capacity hot loop [J/K]"; capc "thermal capacity cold loop [J/K]"; UA "heat loss coefficient [W/K]"
      mask help:
      | Linearized heat pump model, uses measured data according to EN 14511 as input (Schwamberger, K.: Fortschrittsberichete VDI, Nr. 263, 1991).
      | heating power: Qdot_h = K1*Tcold_in + K2*Thot_out + K3
      | electric power: Pel = K4*Tcold_in + K5*Thot_out + K6
      | source power: Qdot_c = -K7*Tcold_in - K8*Thot_out - K9
      | differential equation: cap*dTh/dt = Qdot + mdot*cp*(T_in-T) + UA*(Tamb-T)
      | with: cap = mass * heat_capactiy
      | See hp_param.m for the parameters K1 to K9.
      mask Help: web(fullfile(path_carnot('help'),'HeatPump_basic.html'),'-helpbrowser')
      mask DialogControl ParameterTabVar0 Prompt: HP Caracteristic
      mask DialogControl ParameterTabVar01 Prompt: Thermal
      mask Display: plot(0,-30,120,130,[30,46,36,46,36,46,30],[40,40,50,60,70,80,80],[70,54,64,54,64,54,64,54,64,54,70],[40,40,44,50,55,60,65,70,75,80,80],[56,45],[95,95],[51,51],[82,95])
  T_source : Outport  VectorParamsAs1DForOutWhenUnconnected=off
  "T_out " : Outport  Port=2  VectorParamsAs1DForOutWhenUnconnected=off
  HPdat : Outport  Port=3  VectorParamsAs1DForOutWhenUnconnected=off
  Real P_Therm : Outport  Port=4  VectorParamsAs1DForOutWhenUnconnected=off
  Main Delta : Outport  Port=5  VectorParamsAs1DForOutWhenUnconnected=off
  wires:
  HeatPump_basic/2(THBload) -> "T_out "/1  "THB_s"
  THBsource/1 -> HeatPump_basic/1(Tin_cold)
  THB_r/1 -> HeatPump_basic/2(Tin_hot)
  Tamb/1 -> HeatPump_basic/3(Tamb)
  Ctrl/1 -> HeatPump_basic/4(Ctrl)
  HeatPump_basic/1(Tsource) -> T_source/1  "THBsource"
  HeatPump_basic/3(HPdat) -> HPdat/1
  HeatPump_basic/4(Real P_Therm) -> Real P_Therm/1
  mdot_cold/1 -> HeatPump_basic/5(mdot_in_cold)
  mdot_hot/1 -> HeatPump_basic/6(mdot_in_hot)
  HeatPump_basic/5(Main Delta) -> Main Delta/1
  Defrost Delta In/1 -> HeatPump_basic/7(Defrost Delta In)

== system Final_Model_Building_2_AirflowAdded/ASHP_Subsystem_Variable/DHW for ASHP Case/Storage_Type_2_CONF ==
  note: upper heat exchanger (backup heater)
  note: pipe connection for DHW
  note: pipe connection for DHW circulation
  Tamb : Inport
  Temp_HX : Inport  Port=2
  THB_dhw : Inport  Port=3
  THB_circ : Inport  Port=4
  Mdot_dhw1 : Inport  Port=5
  Mdot_dhw2 : Inport  Port=6
  mdotHEX : Inport  Port=7
  HX_EN12977_1 : Subsystem  AncestorBlock=carnot/Storage/Thermal/Storage_Ports/HX_EN12977  mask(heat exchanger for storage, data EN 12977){h_in=hx1inlet, h_out=hx1outlet, hgt=hgt, dia=hx1dia, height=-0.68756, ua0=hx1uac, uam=hx1uam, uat=hx1uat, dpqua=hx1dpqua, nodes=nodes}
      mask prompts: h_in "relative height of inlet"; h_out "relative height of outlet"; hgt "Height of storage in m"; dia "Diameter of HX pipe [m]"; height "Height difference inlet-outlet [m]"; ua0 "uac: heat transfer coefficient [W/K /(kg/s) /(°C)]"; uam "uam: massflow dependent heat transfer [-]"; uat "uat: temperature difference dependent heat transfer [-]"; dpqua "Pressure drop coefficient dpqua [Pa/(kg/s)²]"; nodes "number of nodes"
      mask help:
      | The block transforms the incoming THV vector to a vector which the storage interprets as a heat exchanger.
      | Give inlet and outlet as a relative position 0=bottom to 1=top
      | The heat transfer is calculated by:
      | UA = uac * mdot^uam * ((Theatexchanger+Tstorage)/2)^uat
      mask init: same as Final_Model_Building_2_AirflowAdded/ASHP_Subsystem/DHW for ASHP Case/Storage_Type_2_CONF/HX_EN12977_1
      mask Help: web(['file:///' fullfile(path_carnot('help'),'StoragePorts_HeatExchangerModels.html')],'-helpbrowser')
      mask TypeOptions dia: Pressure_Drop_StorageHX/dia
      mask TypeOptions height: Pressure_Drop_StorageHX/hgt
      mask TypeOptions ua0: sfun_storage_heatexchanger/p1
      mask TypeOptions uam: sfun_storage_heatexchanger/p2
      mask TypeOptions uat: sfun_storage_heatexchanger/p3
      mask TypeOptions dpqua: Pressure_Drop_StorageHX/dpqua
      mask TypeOptions nodes: sfun_storage_heatexchanger/nodes
      mask DialogControl ParameterTabVar0 Prompt: Geometry
      mask DialogControl ParameterTabVar01 Prompt: Heat transfer
      mask DialogControl ParameterTabVar012 Prompt: Pressure drop
      mask DialogControl ParameterTabVar0123 Prompt: Calculation
      mask Display: disp('HX EN12977')
  Mux : Mux  Inputs=2
  Mux1 : Mux  Inputs=2
  Pipe_Connection_1 : Subsystem  AncestorBlock=carnot/Storage/Thermal/Storage_Ports/Pipe_Connection  mask(pipe connection to storage){h_in=pipe1inlet, h_out=pipe1outlet, hgt=hgt, nodes=nodes}
      mask prompts: h_in "relative height of inlet, range from 0 (= bottom) to 1 (= top)"; h_out "relative height of outlet, range from 0 (= bottom) to 1 (= top)"; hgt "Height of storage in m"; nodes "Number of nodes of storage (DO NOT CHANGE)"
      mask help: The block transforms the incoming THV vector to a vector which the storage interprets as a flow into the storage fluid.
      mask init: same as Final_Model_Building_2_AirflowAdded/ASHP_Subsystem/DHW for ASHP Case/Storage_Type_2_CONF/Pipe_Connection_1
      mask Help: web(fullfile(path_carnot('help'),'StoragePorts_PipeConnections.html'),'-helpbrowser')
      mask DialogControl ParameterTabVar0 Prompt: Geometry
      mask DialogControl ParameterTabVar02 Prompt: Calulation
      mask Display: disp('Pipe')
  Pipe_Connection_2 : Subsystem  AncestorBlock=carnot/Storage/Thermal/Storage_Ports/Pipe_Connection  mask(pipe connection to storage){h_in=pipe2inlet, h_out=pipe2outlet, hgt=hgt, nodes=nodes}
      mask prompts: h_in "relative height of inlet, range from 0 (= bottom) to 1 (= top)"; h_out "relative height of outlet, range from 0 (= bottom) to 1 (= top)"; hgt "Height of storage in m"; nodes "Number of nodes of storage (DO NOT CHANGE)"
      mask help: The block transforms the incoming THV vector to a vector which the storage interprets as a flow into the storage fluid.
      mask init: same as Final_Model_Building_2_AirflowAdded/ASHP_Subsystem/DHW for ASHP Case/Storage_Type_2_CONF/Pipe_Connection_1
      mask Help: web(fullfile(path_carnot('help'),'StoragePorts_PipeConnections.html'),'-helpbrowser')
      mask DialogControl ParameterTabVar0 Prompt: Geometry
      mask DialogControl ParameterTabVar02 Prompt: Calulation
      mask Display: disp('Pipe')
  Scope : Scope
  Scope1 : Scope
  Scope2 : Scope
  T_Sensor_Surface : carnot/Control/T_Sensor_Surface  pos=Tsensor  tdel=10  t0=mean(tini)
      settings: SourceProductName=Carnot
  Terminator1 : Terminator
  sfun_storageTnodesjh : S-Function  AncestorBlock=carnot/Basic/Thermal_Models/sfun_storageTnodes  FunctionName=storage_TnodesMOD  Parameters=dia, volume, standing, uloss , ubot, utop, cond, tini, nodes, nconnect, elimthermocline, condinvtc  SFunctionDeploymentMode=off  EnableBusSupport=off  SFcnStateName=DWORK_DH,DWORK_HCON,DWORK_FLUID,DWORK_MIX,DWORK_PRESS,DWORK_V_NODE,DWORK_LOSS,DWORK_CP_NODE,DWORK_RHO_NODE,DWORK_MDOTIN,DWORK_MDOTUP,DWORK_MDOTDOWN,DWORK_QDOTIN,DWORK_TIN,DWORK_CHK_FLU  mask(sfunction storage_Tnodes){uloss=uwall, ubot=ubot, utop=utop, cond=axcond, volume=volume, dia=dia, standing=standing cylinder, tini=tini, nodes=nodes, nconnect=3, elimthermocline=1, condinvtc=1e5}
      mask prompts: uloss "Heat transfer coefficient to ambient [W/m²K]"; ubot "Heat transfer coefficient to ambient bottom [W/m²K]"; utop "Heat transfer coefficient to ambient top [W/m²K]"; cond "Effective thermal conductivity [W/m/K]"; volume "Volume [m³]"; dia "Diameter [m]"; standing "Position"; tini "Initial temperature in °C"; nodes "Number of nodes"; nconnect "Number of ports"; elimthermocline "Elimination method (0 = off, 1 = temperature dependant, 2 = density dependant)"; condinvtc "COND_ITC: heat transport coefficient for the method 2"
      mask help:
      | The differential equation is derived from the energy conservation equation by using the finite volume method [Patankar: Numerical Heat Transfer and Fluid Flow, 1980].
      | Methods to eliminate the inversed thermocline (It occurs when node with lower density is below a node with higher density. Typically it can be translated to a node with higher temperature below a node with lower temperature. Exception is water below 4°C.):
      | 0 - inversed thermocline is not eliminated
      | 1 - Temperature based: An inversed thermocline exists , if the  temperature of the lower node is more than LIMIT_T_INVERSED degrees  above the upper node. In that case the temperatures of the nodes are mixed. For the geometry of a laying cylinder the different volumes of the nodes are taken in account.
      |  2 - Density based : An inversed thermocline exists, if the density of the lower node is less than the density of the upper node. The model  adds an additional heat transport towards the upper node:
      | heat transport [W/m³] = COND_ITC[W*m³/kg] * density_differnce[kg/m³] / node[m³]
      mask init: same as Final_Model_Building_2_AirflowAdded/ASHP_Subsystem/DHW for ASHP Case/Storage_Type_2_CONF/sfun_storageTnodesjh
      settings: SFcnIsStateOwnerBlock=on
      mask Help: web(fullfile(path_carnot('help'),'Storage_Type_N.html'),'-helpbrowser')
      mask TypeOptions standing: standing cylinder | lying cylinder
      mask DialogControl Container5 Prompt: Thermal
      mask DialogControl Container6 Prompt: Geometry
      mask DialogControl Container7 Prompt: Caclulation
      mask DialogControl Container10 Prompt: Inversed thermocline
      mask Display:
      | disp('storage_Tnodes')
      | 
      | port_label('input', 1, 'Tamb')
      | port_label('output', 1, 'Energy')
      | port_label('output', 2, 'Tnodes')
      | 
      | if exist('nconnect','var')
      |     for n = 1:nconnect
      |         port_label('input',  n+1, ['port' num2str(n)])
      |     end
      | end
  Tsensors : Outport  VectorParamsAs1DForOutWhenUnconnected=off
  THB_hx : Outport  Port=2  VectorParamsAs1DForOutWhenUnconnected=off
  THBdhw : Outport  Port=3  VectorParamsAs1DForOutWhenUnconnected=off
  AuxHeat : Outport  Port=4  VectorParamsAs1DForOutWhenUnconnected=off
  wires:
  HX_EN12977_1/1(to_storeT) -> sfun_storageTnodesjh/4
  Pipe_Connection_2/1(to_storeT) -> Scope/1, sfun_storageTnodesjh/3
  THB_circ/1 -> Mux1/1  "THBinPipe2"
  Tamb/1 -> sfun_storageTnodesjh/1  "Tamb"
  sfun_storageTnodesjh/2 -> Scope2/1, T_Sensor_Surface/1, HX_EN12977_1/1(from_storeT)  "Tnodes"
  Pipe_Connection_1/1(to_storeT) -> THBdhw/1, sfun_storageTnodesjh/2, Scope1/1
  Temp_HX/1 -> HX_EN12977_1/2(Tempin)
  HX_EN12977_1/2(TempHEXout) -> THB_hx/1
  T_Sensor_Surface/1 -> Tsensors/1
  Mdot_dhw1/1 -> Mux/2  "THBinPipe1"
  sfun_storageTnodesjh/1 -> Terminator1/1  "Energy"
  Mdot_dhw2/1 -> Mux1/2  "THBinPipe1"
  THB_dhw/1 -> Mux/1  "THBinPipe1"
  Mux/1 -> Pipe_Connection_1/1(THBin)
  Mux1/1 -> Pipe_Connection_2/1(THBin)
  mdotHEX/1 -> HX_EN12977_1/3(massFlowIn)
  HX_EN12977_1/3(AuxHeat) -> AuxHeat/1

== system Final_Model_Building_2_AirflowAdded/ASHP_Subsystem_Variable/DHW for ASHP Case/Subsystem ==
  In1 : Inport
  Ceil : Rounding
  Constant1 : Constant  Value=60
  Constant2 : Constant  Value=60
  Digital Clock : DigitalClock  SampleTime=10
  Direct Lookup Table (n-D) : LookupNDDirect  NumberOfTableDimensions=1  TableIsInput=on
  Divide : Product  Inputs=*/
  Divide1 : Product  Inputs=*/
  Saturation : Saturate  UpperLimit=1440*365  LowerLimit=0
  Out1 : Outport  VectorParamsAs1DForOutWhenUnconnected=off
  wires:
  Divide1/1 -> Direct Lookup Table (n-D)/2
  Divide/1 -> Ceil/1
  Digital Clock/1 -> Divide/1
  Constant1/1 -> Divide/2
  In1/1 -> Divide1/1
  Direct Lookup Table (n-D)/1 -> Out1/1
  Constant2/1 -> Divide1/2
  Ceil/1 -> Saturation/1
  Saturation/1 -> Direct Lookup Table (n-D)/1

== system Final_Model_Building_2_AirflowAdded/ASHP_Subsystem_Variable/DHW for ASHP Case/Switch Case Action Subsystem ==
  In1 : Inport
  Action Port : ActionPort  ActionPortLabel=default:
  1 m : Relay  OnSwitchValue=Tank_Upper_Temp  OffSwitchValue=Tank_Lower_Temp  OnOutputValue=0  OffOutputValue=1  OutDataTypeStr=boolean
  Out1 : Outport  VectorParamsAs1DForOutWhenUnconnected=off
  wires:
  In1/1 -> 1 m/1
  1 m/1 -> Out1/1

== system Final_Model_Building_2_AirflowAdded/ASHP_Subsystem_Variable/DHW for ASHP Case/Switch Case Action Subsystem1 ==
  In1 : Inport
  Action Port : ActionPort  ActionPortLabel=case [ 0 ]:
  'Aux Required' Alternative1 : Relay  OnSwitchValue=Aux_Threshold  OffSwitchValue=Aux_Threshold-0.1  OnOutputValue=0  OffOutputValue=1  OutDataTypeStr=boolean
  Out1 : Outport  VectorParamsAs1DForOutWhenUnconnected=off
  wires:
  In1/1 -> 'Aux Required' Alternative1/1
  'Aux Required' Alternative1/1 -> Out1/1

== system Final_Model_Building_2_AirflowAdded/ASHP_Subsystem_Variable/DHW for ASHP Case/Switch Case Action Subsystem2 ==
  In1 : Inport
  Action Port : ActionPort  ActionPortLabel=default:
  1 means tank temp recently fell below 49.1 : Relay  OnSwitchValue=60  OffSwitchValue=49.5  OnOutputValue=0  OffOutputValue=1  OutDataTypeStr=boolean
  Out1 : Outport  VectorParamsAs1DForOutWhenUnconnected=off
  wires:
  In1/1 -> 1 means tank temp recently fell below 49.1/1
  1 means tank temp recently fell below 49.1/1 -> Out1/1

== system Final_Model_Building_2_AirflowAdded/ASHP_Subsystem_Variable/DHW for ASHP Case/Switch Case Action Subsystem3 ==
  In1 : Inport
  Action Port : ActionPort  ActionPortLabel=case [ 0 ]:
  'Aux Required' Alternative : Relay  OnSwitchValue=60  OffSwitchValue=Aux_Threshold  OnOutputValue=0  OffOutputValue=1  OutDataTypeStr=boolean
  Out1 : Outport  VectorParamsAs1DForOutWhenUnconnected=off
  wires:
  In1/1 -> 'Aux Required' Alternative/1
  'Aux Required' Alternative/1 -> Out1/1

== system Final_Model_Building_2_AirflowAdded/ASHP_Subsystem_Variable/Defrost Timer/Subsystem ==
  In1 : Inport
  In2 : Inport  Port=2
  1-D Lookup Table : Lookup_n-D  NumberOfTableDimensions=1  BreakpointsForDimension1=[-9.9 1.69 1.71 10]  Table=[0.1833 0.1157 0 0]  InternalRulePriority=Speed  RndMeth=Simplest
  Add One seconds worth of half an hour : Constant
  Add Zero : Constant  Value=0
  Add Zero1 : Constant  Value=10
  Add Zero2 : Constant  Value=0
  Display : Display
  Divide : Product  Inputs=*/
  Divide1 : Product  Inputs=**
  Do Nothing : Constant  Value=0
  Integrator : Integrator  ExternalReset=rising  ShowStatePort=on
  Integrator1 : Integrator  ExternalReset=rising
  Logical Operator : Logic  AllPortsSameDT=off  OutDataTypeStr=boolean
  Relational Operator : RelationalOperator  Operator=<=  OutDataTypeStr=boolean  RndMeth=Simplest  InputSameDT=off
  Reset Integrator : Constant
  Reset Integrator1 : Constant
  Sample and Hold : dspsigops/Sample and Hold  trig=Rising edge  initCond=240  latchinput=on
  Scope1 : Scope
  Scope2 : Scope
  Scope3 : Scope
  Switch{,1..3} (4 alike) : Switch  Threshold=1  SaturateOnIntegerOverflow=off  InputSameDT=off
  Temperature2 : Constant  Value=1.7
  minutes of cold operation before defrost : Constant  Value=Defrost_After_Time
  seconds in 1 min : Constant  Value=60
  Out1 : Outport  VectorParamsAs1DForOutWhenUnconnected=off
  Out2 : Outport  Port=2  VectorParamsAs1DForOutWhenUnconnected=off
  Out3 : Outport  Port=3  VectorParamsAs1DForOutWhenUnconnected=off
  wires:
  In1/1 -> Switch2/1, Relational Operator/1
  Integrator/State -> Switch1/2
  In2/1 -> Switch3/2
  Relational Operator/1 -> Logical Operator/1
  Integrator1/1 -> Sample and Hold/1, Scope1/1
  Switch1/1 -> Integrator/2, Scope3/1, Out1/1, Sample and Hold/Trigger, Integrator1/2
  Switch2/1 -> 1-D Lookup Table/1
  Add One seconds worth of half an hour/1 -> Divide/1
  Integrator/1 -> Scope2/1, Out3/1, Display/1
  Temperature2/1 -> Relational Operator/2
  Switch/1 -> Integrator/1
  Add Zero1/1 -> Switch2/3
  Reset Integrator1/1 -> Switch3/1
  Do Nothing/1 -> Switch1/3
  Logical Operator/1 -> Switch/2, Switch2/2
  Switch3/1 -> Logical Operator/2
  Add Zero2/1 -> Switch3/3
  Reset Integrator/1 -> Switch1/1
  Add Zero/1 -> Switch/3
  1-D Lookup Table/1 -> Integrator1/1
  Sample and Hold/1 -> Out2/1
  Divide1/1 -> Divide/2
  Divide/1 -> Switch/1
  seconds in 1 min/1 -> Divide1/2
  minutes of cold operation before defrost/1 -> Divide1/1

== system Final_Model_Building_2_AirflowAdded/ASHP_Subsystem_Variable/Defrost Timer/Subsystem1 ==
  In1 : Inport
  In2 : Inport  Port=2
  In3 : Inport  Port=3
  Counter On? (i.e. not currently defrosting?)1 : Constant  Value=0
  Counter On? (i.e. not currently defrosting?)3 : Constant  Value=20
  Discrete-Time Integrator : DiscreteIntegrator  gainval=1  ExternalReset=rising  SampleTime=-1  ICPrevOutput=DiscIntNeverNeededParam  ICPrevScaledInput=DiscIntNeverNeededParam
  Integrator1 : Integrator  ExternalReset=rising  ShowStatePort=on
  Product : Product  Inputs=*/
  Product2 : Product
  Saturation : Saturate  UpperLimit=1  LowerLimit=0
  Switch : Switch  Threshold=1  SaturateOnIntegerOverflow=off  InputSameDT=off
  Terminator : Terminator
  Terminator1 : Terminator
  "d " : Constant
  Out1 : Outport  VectorParamsAs1DForOutWhenUnconnected=off
  wires:
  "d "/1 -> Switch/1
  Product/1 -> Switch/2
  Discrete-Time Integrator/1 -> Product2/1
  Switch/1 -> Discrete-Time Integrator/2, Integrator1/2
  Counter On? (i.e. not currently defrosting?)1/1 -> Switch/3
  In2/1 -> Product/2
  In1/1 -> Discrete-Time Integrator/1
  Counter On? (i.e. not currently defrosting?)3/1 -> Product2/2
  Product2/1 -> Saturation/1
  Saturation/1 -> Out1/1, Integrator1/1
  Integrator1/State -> Product/1
  Integrator1/1 -> Terminator/1
  In3/1 -> Terminator1/1
